simulink model "PosControl_Sim"  (R2017b)
settings: Solver=ode4  StartTime=0.0  StopTime=2  FixedStep=0.001  RelTol=1e-3
InitFcn:
  | Init_control;
values from neighbouring files (symbols this model uses):
  DEG2RAD = 0.0174533    [Init_control.m]
  Kd_PITCH_AngleRate = 0.001    [Init_control.m]
  Kd_ROLL_AngleRate = 0.001    [Init_control.m]
  Kd_YAW_AngleRate = 0.00    (= 0)    [Init_control.m]
  Ki_PITCH_AngleRate = 0.02    [Init_control.m]
  Ki_ROLL_AngleRate = 0.02    [Init_control.m]
  Ki_YAW_AngleRate = 0.01    [Init_control.m]
  Kp_PITCH_ANGLE = 6.5    [Init_control.m]
  Kp_PITCH_AngleRate = 0.1    [Init_control.m]
  Kp_ROLL_ANGLE = 6.5    [Init_control.m]
  Kp_ROLL_AngleRate = 0.1    [Init_control.m]
  Kp_YAW_AngleRate = 0.5    [Init_control.m]
  Kpxp = 1.0    (= 1)    [Init_control.m]
  Kpyp = 1.0    (= 1)    [Init_control.m]
  Kpzp = 4.0    (= 4)    [Init_control.m]
  Kvxd = 0.01    [Init_control.m]
  Kvxi = 0.4    [Init_control.m]
  Kvxp = 2.5    [Init_control.m]
  Kvyd = 0.01    [Init_control.m]
  Kvyi = 0.4    [Init_control.m]
  Kvyp = 2.5    [Init_control.m]
  Kvzd = 0.005    [Init_control.m]
  Kvzi = 0.01    [Init_control.m]
  Kvzp = 0.45    [Init_control.m]
  MAX_CONTROL_ANGLE_PITCH = 35    [Init_control.m]
  MAX_CONTROL_ANGLE_RATE_PITCH = 220    [Init_control.m]
  MAX_CONTROL_ANGLE_RATE_ROLL = 220    [Init_control.m]
  MAX_CONTROL_ANGLE_RATE_Y = 200    [Init_control.m]
  MAX_CONTROL_ANGLE_ROLL = 35    [Init_control.m]
  MAX_CONTROL_VELOCITY_XY = 5    [Init_control.m]
  MAX_CONTROL_VELOCITY_Z = 3    [Init_control.m]
  ModelInit_AngEuler = [0, 0, 0]    [Init_control.m]
  ModelInit_PosE = [0, 0, -100]    [Init_control.m]
  ModelInit_Rads = 0    [Init_control.m]
  ModelInit_RateB = [0, 0, 0]    [Init_control.m]
  ModelInit_VelB = [0, 0, 0]    [Init_control.m]
  Saturation_I_ah = 3.43    [Init_control.m]
  Saturation_I_az = 5    [Init_control.m]
  Saturation_I_RP_Max = 0.3    [Init_control.m]
  Saturation_I_RP_Min = -0.3    [Init_control.m]
  Saturation_I_Y_Max = 0.2    [Init_control.m]
  Saturation_I_Y_Min = -0.2    [Init_control.m]
  THR_HOVER = 0.609    [Init_control.m]
undefined symbols (not defined in the file or in its folder): DiscIntNeverNeededParam, earthRadius, ModelParam_envGravityAcc, ModelParam_motorCr, ModelParam_motorJm, ModelParam_motorT, ModelParam_motorWb, ModelParam_rotorCm, ModelParam_rotorCt, ModelParam_uavCCm, ModelParam_uavCd, ModelParam_uavJ, ModelParam_uavMass, ModelParam_uavR, Receive, Send
libraries: simulink x8, aerolibfltsims x3, sharedutil x2, aerolibanimutils x1
(part 1 of 2)
settings Model: Creator=wsh  LastModifiedBy=Mr Wang
settings DebuggingCC: BusObjectLabelMismatch=error
settings CodeAppCC: StateflowObjectComments=on

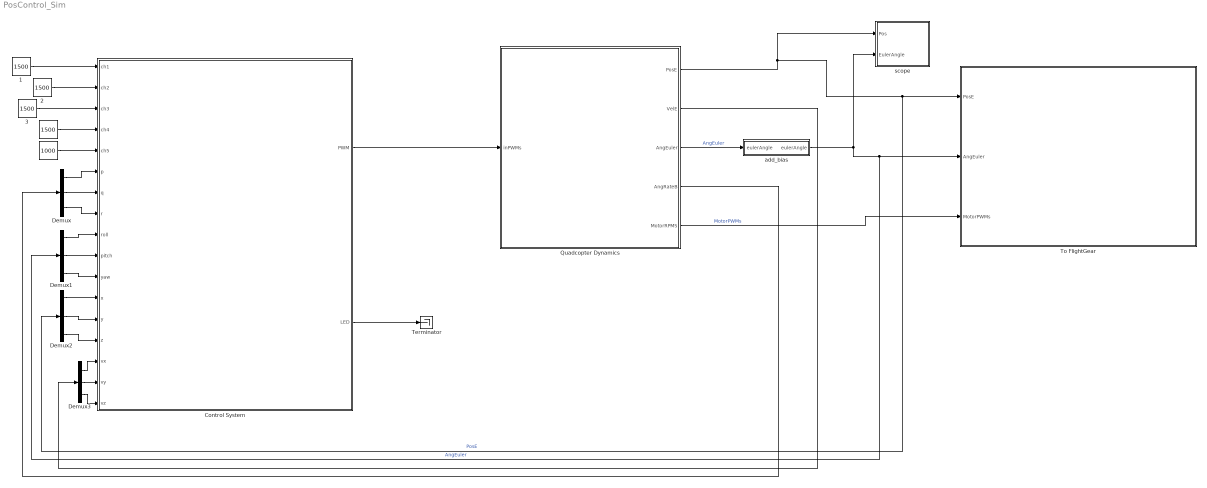
== system PosControl_Sim ==
  " " : Constant  Value=1000  OutDataTypeStr=uint16
  "          " : Constant  Value=1500  OutDataTypeStr=uint16
  "   1" : Constant  Value=1500  OutDataTypeStr=uint16
  "   2" : Constant  Value=1500  OutDataTypeStr=uint16
  "   3" : Constant  Value=1500  OutDataTypeStr=uint16
  Control System : Subsystem
      mask Display: image('icon\pixhawk.png');
  Demux{,1..3} (4 alike) : Demux  Outputs=3
  Quadcopter Dynamics : Subsystem
      mask Display: image('./icon/F450.png');
  Terminator : Terminator
  To FlightGear : Subsystem
      mask Display: image('./icon/FlightGear.png');
  add_bias : Subsystem
  scope : Subsystem
  wires:
  Quadcopter Dynamics/1(PosE) -> scope/1(Pos), To FlightGear/1(PosE), Demux2/1  "PosE"
  Quadcopter Dynamics/5(MotorRPMS) -> To FlightGear/3(MotorPWMs)  "MotorPWMs"
  Control System/2(LED) -> Terminator/1
  add_bias/1("eulerAngle ") -> scope/2(EulerAngle), To FlightGear/2(AngEuler), Demux1/1  "AngEuler"
  "          "/1 -> Control System/4(ch4)
  Quadcopter Dynamics/4(AngRateB) -> Demux/1
  " "/1 -> Control System/5(ch5)
  Demux/1 -> Control System/6(p)
  Demux/2 -> Control System/7(q)
  Demux/3 -> Control System/8(r)
  Demux2/1 -> Control System/12(x)
  Demux2/2 -> Control System/13(y)
  Demux2/3 -> Control System/14(z)
  Demux3/1 -> Control System/15(vx)
  Demux3/2 -> Control System/16(vy)
  Demux3/3 -> Control System/17(vz)
  "   1"/1 -> Control System/1(ch1)
  Quadcopter Dynamics/2(VelE) -> Demux3/1
  "   2"/1 -> Control System/2(ch2)
  Quadcopter Dynamics/3(AngEuler) -> add_bias/1(eulerAngle)  "AngEuler"
  Demux1/2 -> Control System/10(pitch)
  Demux1/1 -> Control System/9(roll)
  Demux1/3 -> Control System/11(yaw)
  "   3"/1 -> Control System/3(ch3)
  Control System/1(PWM) -> Quadcopter Dynamics/1(inPWMs)

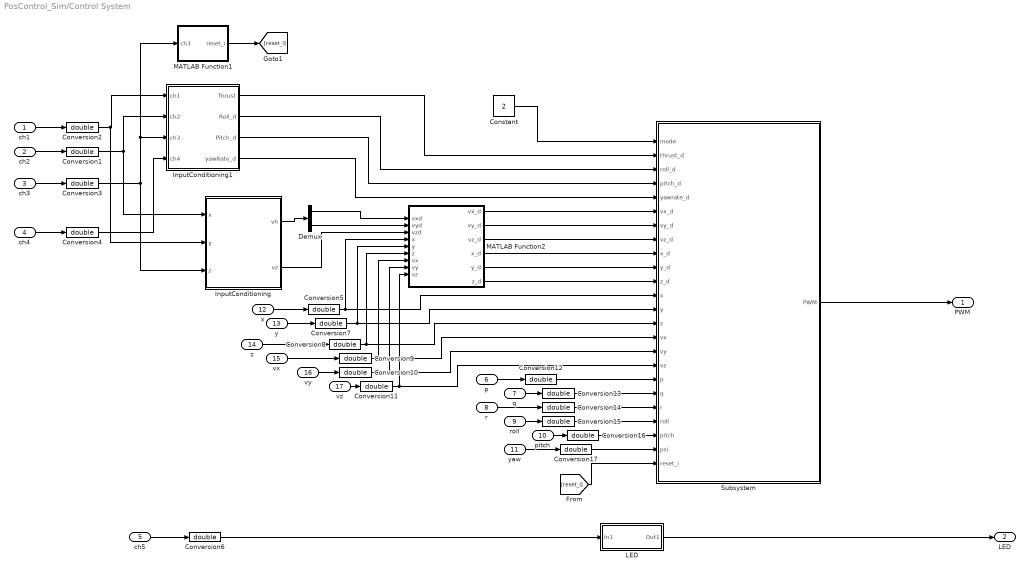
== system PosControl_Sim/Control System ==
  ch1 : Inport  OutDataTypeStr=uint16  PortDimensions=1
  ch2 : Inport  Port=2  OutDataTypeStr=uint16  PortDimensions=1
  ch3 : Inport  Port=3  OutDataTypeStr=uint16  PortDimensions=1
  ch4 : Inport  Port=4  OutDataTypeStr=uint16  PortDimensions=1
  ch5 : Inport  Port=5  OutDataTypeStr=uint16  PortDimensions=1  Interpolate=off
  p : Inport  Port=6  PortDimensions=1
  q : Inport  Port=7  PortDimensions=1
  r : Inport  Port=8  PortDimensions=1
  roll : Inport  Port=9  PortDimensions=1
  pitch : Inport  Port=10  PortDimensions=1
  yaw : Inport  Port=11  PortDimensions=1
  x : Inport  Port=12
  y : Inport  Port=13
  z : Inport  Port=14
  vx : Inport  Port=15
  vy : Inport  Port=16
  vz : Inport  Port=17
  Constant : Constant  Value=2
  Conversion{1..17} (17 alike) : DataTypeConversion  OutDataTypeStr=double
  Demux : Demux  Outputs=2
  InputConditioning : Subsystem
  InputConditioning1 : Subsystem
  "LED " : Subsystem
  MATLAB Function1 : MATLAB Function  TreatAsAtomicUnit=on
  MATLAB Function2 : MATLAB Function  TreatAsAtomicUnit=on
  Subsystem : Subsystem
  PWM : Outport
  LED : Outport  Port=2  PortDimensions=1
  wires:
  ch3/1 -> Conversion3/1
  ch5/1 -> Conversion6/1
  ch4/1 -> Conversion4/1
  "LED "/1(Out1) -> LED/1
  Conversion6/1 -> "LED "/1(In1)
  Conversion4/1 -> InputConditioning1/4(ch4)
  ch1/1 -> Conversion2/1
  ch2/1 -> Conversion1/1
  Conversion1/1 -> InputConditioning/1(x), InputConditioning1/2(ch2)
  x/1 -> Conversion5/1
  y/1 -> Conversion7/1
  z/1 -> Conversion8/1
  Constant/1 -> Subsystem/1(mode)
  roll/1 -> Conversion15/1
  pitch/1 -> Conversion16/1
  p/1 -> Conversion12/1
  q/1 -> Conversion13/1
  r/1 -> Conversion14/1
  yaw/1 -> Conversion17/1
  vz/1 -> Conversion11/1
  vy/1 -> Conversion10/1
  vx/1 -> Conversion9/1
  InputConditioning1/2(Roll_d) -> Subsystem/3(roll_d)
  InputConditioning1/3(Pitch_d) -> Subsystem/4(pitch_d)
  InputConditioning1/1(Thrust) -> Subsystem/2(thrust_d)
  InputConditioning1/4(yawRate_d) -> Subsystem/5(yawrate_d)
  Conversion5/1 -> Subsystem/12(x), MATLAB Function2/4(x)
  Conversion7/1 -> Subsystem/13(y), MATLAB Function2/5(y)
  Conversion8/1 -> Subsystem/14(z), MATLAB Function2/6(z)
  Conversion9/1 -> Subsystem/15(vx), MATLAB Function2/7(vx)
  Conversion10/1 -> Subsystem/16(vy), MATLAB Function2/8(vy)
  Conversion11/1 -> Subsystem/17(vz), MATLAB Function2/9(vz)
  Conversion12/1 -> Subsystem/18(p)
  Conversion13/1 -> Subsystem/19(q)
  Conversion14/1 -> Subsystem/20(r)
  Conversion15/1 -> Subsystem/21(roll)
  Conversion16/1 -> Subsystem/22(pitch)
  Conversion17/1 -> Subsystem/23(psi)
  Conversion3/1 -> InputConditioning/3(z), InputConditioning1/3(ch3), MATLAB Function1/1(ch3)
  MATLAB Function1/1(reset_i) -> [reset_i]
  [reset_i] -> Subsystem/24(reset_i)
  Conversion2/1 -> InputConditioning/2(y), InputConditioning1/1("ch1 ")
  InputConditioning/2(vz) -> MATLAB Function2/3(vzd)
  MATLAB Function2/1(vx_d) -> Subsystem/6(vx_d)
  MATLAB Function2/2(vy_d) -> Subsystem/7(vy_d)
  MATLAB Function2/3(vz_d) -> Subsystem/8(vz_d)
  MATLAB Function2/4(x_d) -> Subsystem/9(x_d)
  MATLAB Function2/5(y_d) -> Subsystem/10(y_d)
  MATLAB Function2/6(z_d) -> Subsystem/11(z_d)
  InputConditioning/1(vh) -> Demux/1
  Demux/1 -> MATLAB Function2/1(vxd)
  Demux/2 -> MATLAB Function2/2(vyd)
  Subsystem/1(PWM) -> PWM/1

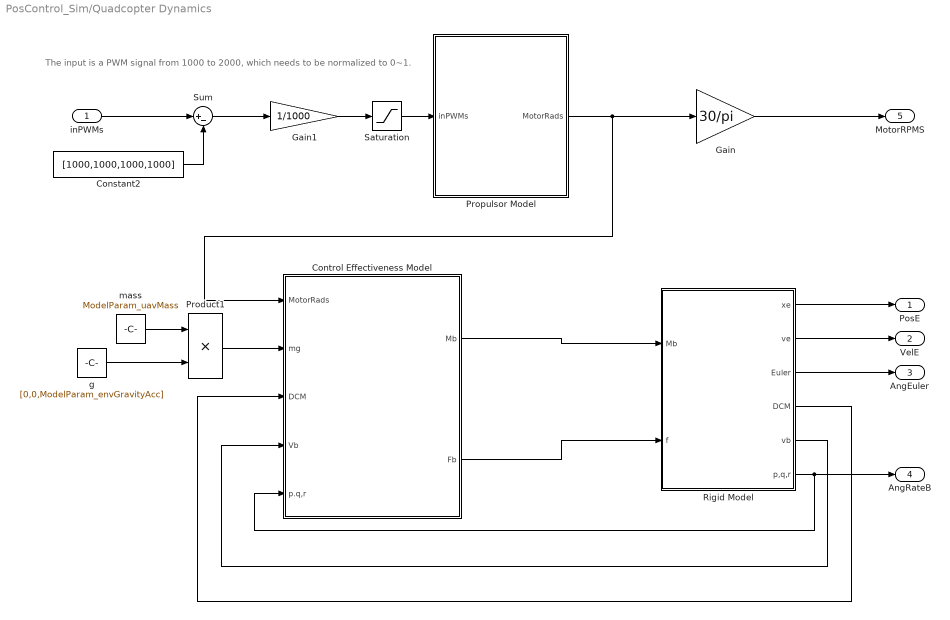
== system PosControl_Sim/Quadcopter Dynamics ==
  note: The input is a PWM signal from 1000 to 2000,
      | which needs to be normalized to 0~1.
  inPWMs : Inport
  Constant2 : Constant  Value=[1000,1000,1000,1000]
  Control Effectiveness Model : Subsystem
  Gain : Gain  Gain=30/pi
  Gain1 : Gain  Gain=1/1000
  Product1 : Product
  Propulsor Model : Subsystem
  Rigid Model : Subsystem
  Saturation : Saturate  UpperLimit=1  LowerLimit=0
  Sum : Sum  Inputs=|+-
  g : Constant  Value=[0,0,ModelParam_envGravityAcc]
  mass : Constant  Value=ModelParam_uavMass
  PosE : Outport
  VelE : Outport  Port=2
  AngEuler : Outport  Port=3
  AngRateB : Outport  Port=4
  MotorRPMS : Outport  Port=5
  wires:
  Saturation/1 -> Propulsor Model/1(inPWMs)
  Rigid Model/6("p,q,r ") -> Control Effectiveness Model/5(p.q,r), AngRateB/1
  mass/1 -> Product1/1
  Rigid Model/4(DCM) -> Control Effectiveness Model/3(DCM)
  Propulsor Model/1(MotorRads) -> Gain/1, Control Effectiveness Model/1(MotorRads)
  Gain1/1 -> Saturation/1
  Rigid Model/2(ve) -> VelE/1
  Sum/1 -> Gain1/1
  Product1/1 -> Control Effectiveness Model/2(mg)
  Rigid Model/5("vb ") -> Control Effectiveness Model/4(Vb)
  Rigid Model/1("xe ") -> PosE/1
  Rigid Model/3(Euler) -> AngEuler/1
  Control Effectiveness Model/1(Mb) -> Rigid Model/1(Mb)
  inPWMs/1 -> Sum/1
  Control Effectiveness Model/2(Fb) -> Rigid Model/2(f)
  Constant2/1 -> Sum/2
  g/1 -> Product1/2
  Gain/1 -> MotorRPMS/1

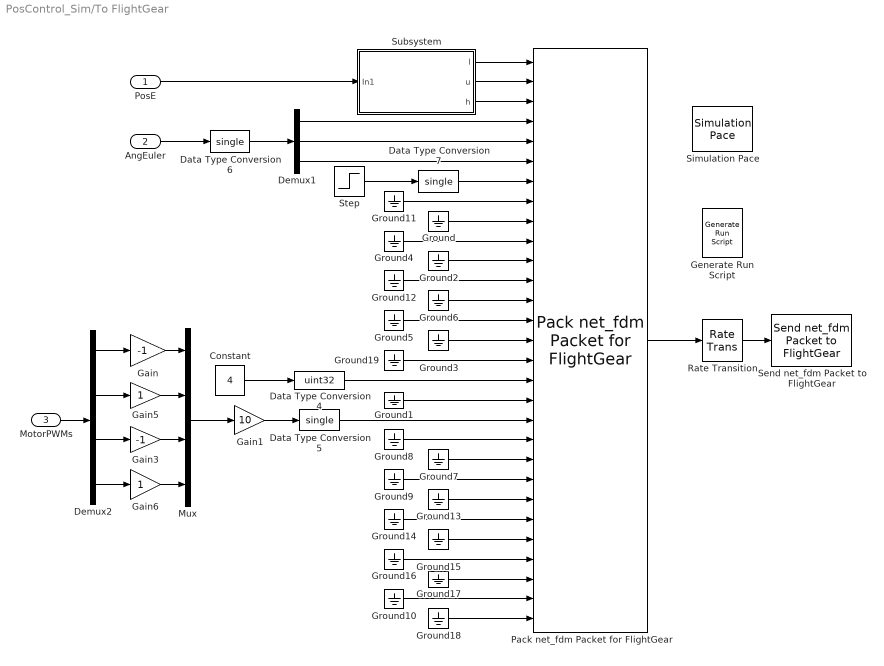
== system PosControl_Sim/To FlightGear ==
  PosE : Inport
  AngEuler : Inport  Port=2
  MotorPWMs : Inport  Port=3
  Constant : Constant  Value=4
  Data Type Conversion4 : DataTypeConversion  OutDataTypeStr=uint32
  Data Type Conversion5 : DataTypeConversion  OutDataTypeStr=single
  Data Type Conversion6 : DataTypeConversion  OutDataTypeStr=single
  Data Type Conversion7 : DataTypeConversion  OutDataTypeStr=single
  Demux1 : Demux  Outputs=3
  Demux2 : Demux
  Gain : Gain  Gain=-1
  Gain1 : Gain  Gain=10
  Gain3 : Gain  Gain=-1
  Gain5 : Gain
  Gain6 : Gain
  Generate Run Script : aerolibfltsims/Generate Run Script  OutputFileName=runfg_myownUAV.bat  FlightGearBaseDirectory=C:\Program Files\FlightGear 2016.1.2  GeometryModelName=myownUAV  DestinationPort=5502  OriginAddress=127.0.0.1  OriginPort=5505  LocalAddress=127.0.0.1  AirportId=KSFO  RunwayId=10L  InitialAltitude=0  InitialHeading=0  OffsetDistance=0  OffsetAzimuth=0  GenerateFile=off  Architecture=Default  dataFlow=Send-Receive
  Ground{,1..19} (20 alike) : Ground
  Mux : Mux
  Pack net_fdm Packet for FlightGear : aerolibfltsims/Pack net_fdm Packet for FlightGear  FlightGearVersion=v2016.1  ShowPositionAttitudeInputs=on  ShowVelocityAccelerationInputs=off  ShowControlSurfacePositionInputs=on  ShowEngineFuelInputs=on  ShowLandingGearInputs=off  ShowEnvironmentInputs=off  SampleTime=0.01
      settings: SourceProductName=Aerospace Blockset  SourceProductBaseCode=AE
  Rate Transition : RateTransition
  Send net_fdm Packet to FlightGear : aerolibfltsims/Send net_fdm Packet to FlightGear  DestinationIpAddress=127.0.0.1  DestinationPort=5502  LocalIpPort=-1  varLen=off  SampleTime=0.005
      settings: SourceProductName=Aerospace Blockset  SourceProductBaseCode=AE
  Simulation Pace : aerolibanimutils/Simulation Pace  SimulationPace=1  SleepMode=MATLAB Thread  OutputPaceError=off  SampleTime=-1
      settings: AttributesFormatString=%<SimulationPace> sec/sec
  Step : Step  Time=0  SampleTime=0
  Subsystem : Subsystem
  wires:
  Gain1/1 -> Data Type Conversion5/1
  Data Type Conversion6/1 -> Demux1/1
  Demux1/3 -> Pack net_fdm Packet for FlightGear/6
  Demux1/2 -> Pack net_fdm Packet for FlightGear/5
  Demux1/1 -> Pack net_fdm Packet for FlightGear/4
  Ground19/1 -> Pack net_fdm Packet for FlightGear/16
  Subsystem/3(h) -> Pack net_fdm Packet for FlightGear/3
  Subsystem/2(u) -> Pack net_fdm Packet for FlightGear/2
  Subsystem/1("l ") -> Pack net_fdm Packet for FlightGear/1
  PosE/1 -> Subsystem/1(In1)
  Rate Transition/1 -> Send net_fdm Packet to FlightGear/1
  Gain6/1 -> Mux/4
  Demux2/4 -> Gain6/1
  Gain5/1 -> Mux/2
  Demux2/2 -> Gain5/1
  Gain3/1 -> Mux/3
  Gain/1 -> Mux/1
  Demux2/3 -> Gain3/1
  Demux2/1 -> Gain/1
  Mux/1 -> Gain1/1
  MotorPWMs/1 -> Demux2/1
  AngEuler/1 -> Data Type Conversion6/1
  Ground12/1 -> Pack net_fdm Packet for FlightGear/12
  Ground2/1 -> Pack net_fdm Packet for FlightGear/11
  Data Type Conversion5/1 -> Pack net_fdm Packet for FlightGear/19
  Constant/1 -> Data Type Conversion4/1
  Ground11/1 -> Pack net_fdm Packet for FlightGear/8
  Ground4/1 -> Pack net_fdm Packet for FlightGear/10
  Ground6/1 -> Pack net_fdm Packet for FlightGear/13
  Ground5/1 -> Pack net_fdm Packet for FlightGear/14
  Ground3/1 -> Pack net_fdm Packet for FlightGear/15
  Ground1/1 -> Pack net_fdm Packet for FlightGear/18
  Data Type Conversion4/1 -> Pack net_fdm Packet for FlightGear/17
  Step/1 -> Data Type Conversion7/1
  Ground18/1 -> Pack net_fdm Packet for FlightGear/29
  Ground10/1 -> Pack net_fdm Packet for FlightGear/28
  Ground17/1 -> Pack net_fdm Packet for FlightGear/27
  Ground16/1 -> Pack net_fdm Packet for FlightGear/26
  Ground15/1 -> Pack net_fdm Packet for FlightGear/25
  Ground14/1 -> Pack net_fdm Packet for FlightGear/24
  Ground13/1 -> Pack net_fdm Packet for FlightGear/23
  Ground9/1 -> Pack net_fdm Packet for FlightGear/22
  Ground7/1 -> Pack net_fdm Packet for FlightGear/21
  Ground/1 -> Pack net_fdm Packet for FlightGear/9
  Ground8/1 -> Pack net_fdm Packet for FlightGear/20
  Data Type Conversion7/1 -> Pack net_fdm Packet for FlightGear/7
  Pack net_fdm Packet for FlightGear/1 -> Rate Transition/1

== system PosControl_Sim/add_bias ==
  eulerAngle : Inport
  Constant : Constant  Value=0.03
  Constant1 : Constant  Value=0.03
  Demux4 : Demux  Outputs=3
  Mux : Mux  Inputs=3
  Sum : Sum  Inputs=|++
  Sum1 : Sum  Inputs=|++
  "eulerAngle " : Outport
  wires:
  Sum/1 -> Mux/1
  eulerAngle/1 -> Demux4/1
  Sum1/1 -> Mux/2
  Demux4/3 -> Mux/3  "yaw"
  Demux4/2 -> Sum1/1  "pitch"
  Constant/1 -> Sum/2
  Demux4/1 -> Sum/1  "roll"
  Constant1/1 -> Sum1/2
  Mux/1 -> "eulerAngle "/1

== system PosControl_Sim/scope ==
  Pos : Inport
  EulerAngle : Inport  Port=2
  Demux1 : Demux  Outputs=3
  Demux4 : Demux  Outputs=3
  Terminator : Terminator
  XY : simulink/Sinks/XY Graph  xmin=-0.2  xmax=3  ymin=-3  ymax=0.2  st=-1
  rp : Scope  NumInputPorts=2
  z : Scope
  wires:
  Demux1/1 -> XY/1
  Demux4/2 -> rp/2
  Demux4/1 -> rp/1
  Demux4/3 -> Terminator/1
  EulerAngle/1 -> Demux4/1
  Pos/1 -> Demux1/1
  Demux1/3 -> z/1
  Demux1/2 -> XY/2

== system PosControl_Sim/Control System/InputConditioning ==
  x : Inport
  y : Inport  Port=2
  z : Inport  Port=3
  Mux21 : Mux  Inputs=2
  Saturation10 : Saturate  UpperLimit=1  LowerLimit=-1
  Saturation8 : Saturate  UpperLimit=1  LowerLimit=-1
  Saturation9 : Saturate  UpperLimit=1  LowerLimit=-1
  deadzone1 : MATLAB Function  TreatAsAtomicUnit=on
  deadzone2 : MATLAB Function  TreatAsAtomicUnit=on
  deadzone3 : MATLAB Function  TreatAsAtomicUnit=on
  max_vx : Gain  Gain=-MAX_CONTROL_VELOCITY_XY  OutDataTypeStr=Inherit: Inherit via back propagation
  max_vy : Gain  Gain=MAX_CONTROL_VELOCITY_XY  OutDataTypeStr=Inherit: Inherit via back propagation
  max_vz : Gain  Gain=-MAX_CONTROL_VELOCITY_Z  OutDataTypeStr=Inherit: Inherit via back propagation
  vh : Outport
  vz : Outport  Port=2
  wires:
  Saturation10/1 -> max_vz/1
  Mux21/1 -> vh/1
  Saturation8/1 -> max_vx/1
  deadzone3/1(y) -> Saturation10/1
  deadzone2/1(y) -> Saturation9/1
  deadzone1/1(y) -> Saturation8/1
  Saturation9/1 -> max_vy/1
  x/1 -> deadzone1/1(u)
  z/1 -> deadzone3/1(u)
  y/1 -> deadzone2/1(u)
  max_vz/1 -> vz/1
  max_vx/1 -> Mux21/1
  max_vy/1 -> Mux21/2

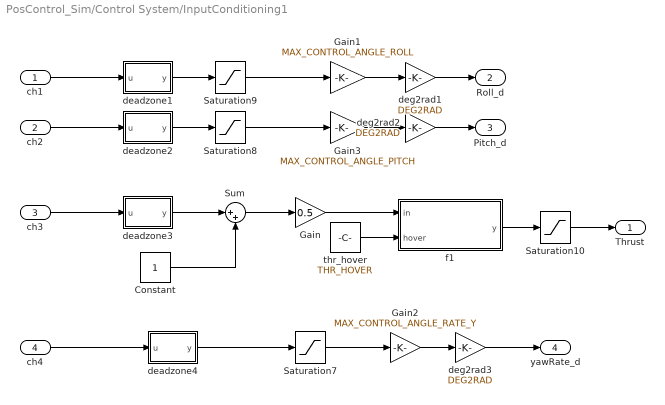
== system PosControl_Sim/Control System/InputConditioning1 ==
  "ch1 " : Inport
  ch2 : Inport  Port=2
  ch3 : Inport  Port=3
  ch4 : Inport  Port=4
  Constant : Constant
  Gain : Gain  Gain=0.5
  Gain1 : Gain  Gain=MAX_CONTROL_ANGLE_ROLL  OutDataTypeStr=Inherit: Inherit via back propagation
  Gain2 : Gain  Gain=MAX_CONTROL_ANGLE_RATE_Y
  Gain3 : Gain  Gain=MAX_CONTROL_ANGLE_PITCH  OutDataTypeStr=Inherit: Inherit via back propagation
  Saturation10 : Saturate  UpperLimit=1  LowerLimit=0
  Saturation7 : Saturate  UpperLimit=1  LowerLimit=-1
  Saturation8 : Saturate  UpperLimit=1  LowerLimit=-1
  Saturation9 : Saturate  UpperLimit=1  LowerLimit=-1
  Sum : Sum  Inputs=|++
  deadzone1 : MATLAB Function  TreatAsAtomicUnit=on
  deadzone2 : MATLAB Function  TreatAsAtomicUnit=on
  deadzone3 : MATLAB Function  TreatAsAtomicUnit=on
  deadzone4 : MATLAB Function  TreatAsAtomicUnit=on
  deg2rad1 : Gain  Gain=DEG2RAD
  deg2rad2 : Gain  Gain=DEG2RAD
  deg2rad3 : Gain  Gain=DEG2RAD
  f1 : MATLAB Function  TreatAsAtomicUnit=on
  "thr_hover " : Constant  Value=THR_HOVER
  Thrust : Outport
  Roll_d : Outport  Port=2
  Pitch_d : Outport  Port=3
  yawRate_d : Outport  Port=4
  wires:
  deadzone3/1(y) -> Sum/1
  ch3/1 -> deadzone3/1(u)
  deadzone2/1(y) -> Saturation8/1
  Saturation10/1 -> Thrust/1
  deadzone1/1(y) -> Saturation9/1
  "ch1 "/1 -> deadzone1/1(u)
  ch2/1 -> deadzone2/1(u)
  Saturation9/1 -> Gain1/1
  Saturation8/1 -> Gain3/1
  Gain3/1 -> deg2rad2/1
  Constant/1 -> Sum/2
  Sum/1 -> Gain/1
  Gain1/1 -> deg2rad1/1
  deg2rad1/1 -> Roll_d/1
  deg2rad2/1 -> Pitch_d/1
  Saturation7/1 -> Gain2/1
  deadzone4/1(y) -> Saturation7/1
  ch4/1 -> deadzone4/1(u)
  Gain2/1 -> deg2rad3/1
  deg2rad3/1 -> yawRate_d/1
  "thr_hover "/1 -> f1/2(hover)
  Gain/1 -> f1/1(in)
  f1/1(y) -> Saturation10/1

== system PosControl_Sim/Control System/LED  ==
  In1 : Inport
  Compare To Constant3 : simulink/Logic and Bit Operations/Compare To Constant  relop=>=  const=uint16(1500)  OutDataTypeStr=boolean
  Out1 : Outport
  wires:
  Compare To Constant3/1 -> Out1/1
  In1/1 -> Compare To Constant3/1

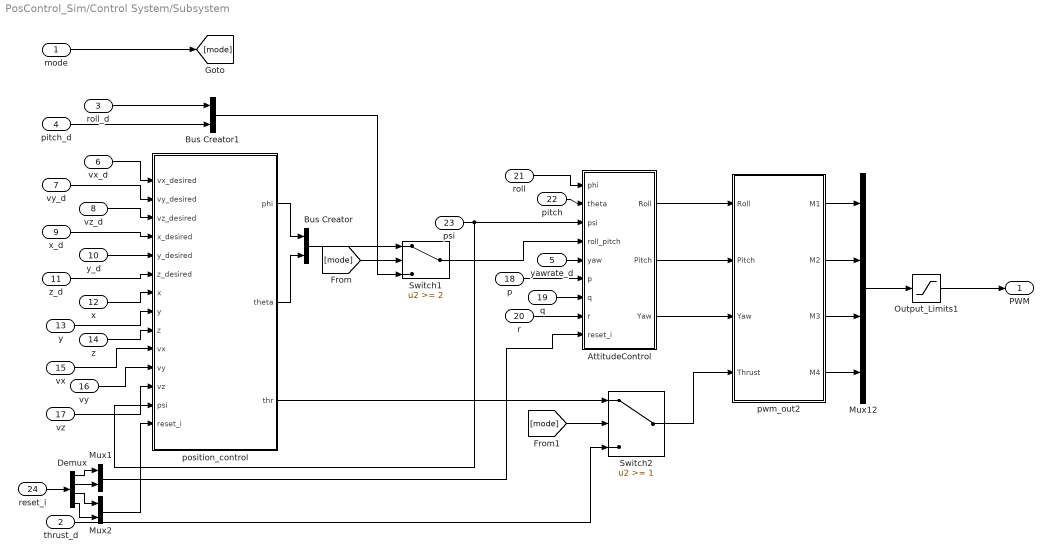
== system PosControl_Sim/Control System/Subsystem ==
  mode : Inport
  thrust_d : Inport  Port=2
  roll_d : Inport  Port=3
  pitch_d : Inport  Port=4
  yawrate_d : Inport  Port=5
  vx_d : Inport  Port=6
  vy_d : Inport  Port=7
  vz_d : Inport  Port=8
  x_d : Inport  Port=9
  y_d : Inport  Port=10
  z_d : Inport  Port=11
  x : Inport  Port=12
  y : Inport  Port=13
  z : Inport  Port=14
  vx : Inport  Port=15
  vy : Inport  Port=16
  vz : Inport  Port=17
  p : Inport  Port=18  PortDimensions=1
  q : Inport  Port=19  PortDimensions=1
  r : Inport  Port=20  PortDimensions=1
  roll : Inport  Port=21  PortDimensions=1
  pitch : Inport  Port=22  PortDimensions=1
  psi : Inport  Port=23  PortDimensions=1
  reset_i : Inport  Port=24
  AttitudeControl : Subsystem
  Bus Creator : BusCreator  Inputs=2
  Bus Creator1 : BusCreator  Inputs=2
  Demux : Demux
  Mux1 : Mux  Inputs=2
  Mux12 : Mux
  Mux2 : Mux  Inputs=2
  Output_Limits1 : Saturate  UpperLimit=2000  LowerLimit=1000
  Switch1 : Switch  Threshold=2
  Switch2 : Switch  Threshold=1
  position_control : Subsystem
  pwm_out2 : MATLAB Function  SystemSampleTime=0.004
  PWM : Outport
  wires:
  pwm_out2/4(M4) -> Mux12/4
  pwm_out2/3(M3) -> Mux12/3
  yawrate_d/1 -> AttitudeControl/5(yaw)
  roll/1 -> AttitudeControl/1(phi)
  Output_Limits1/1 -> PWM/1
  q/1 -> AttitudeControl/7(q)
  AttitudeControl/1(Roll) -> pwm_out2/1(Roll)
  pwm_out2/2(M2) -> Mux12/2
  AttitudeControl/2(Pitch) -> pwm_out2/2(Pitch)
  pitch/1 -> AttitudeControl/2(theta)
  Mux12/1 -> Output_Limits1/1
  position_control/2(theta) -> Bus Creator/2
  pwm_out2/1(M1) -> Mux12/1
  AttitudeControl/3(Yaw) -> pwm_out2/3(Yaw)
  position_control/1(phi) -> Bus Creator/1
  p/1 -> AttitudeControl/6(p)
  vx/1 -> position_control/10(vx)
  vz/1 -> position_control/12(vz)
  vy/1 -> position_control/11(vy)
  x_d/1 -> position_control/4(x_desired)
  y_d/1 -> position_control/5(y_desired)
  z_d/1 -> position_control/6(z_desired)
  mode/1 -> [mode]
  vz_d/1 -> position_control/3(vz_desired)
  x/1 -> position_control/7(x)
  vx_d/1 -> position_control/1(vx_desired)
  vy_d/1 -> position_control/2(vy_desired)
  y/1 -> position_control/8(y)
  z/1 -> position_control/9(z)
  Bus Creator/1 -> Switch1/1
  [mode] -> Switch1/2
  Switch1/1 -> AttitudeControl/4(roll_pitch)
  roll_d/1 -> Bus Creator1/1
  pitch_d/1 -> Bus Creator1/2
  Bus Creator1/1 -> Switch1/3
  [mode] -> Switch2/2
  position_control/3(thr) -> Switch2/1
  Switch2/1 -> pwm_out2/4(Thrust)
  thrust_d/1 -> Switch2/3
  r/1 -> AttitudeControl/8(r)
  psi/1 -> AttitudeControl/3(psi), position_control/13(psi)
  reset_i/1 -> Demux/1
  Mux2/1 -> position_control/14(reset_i)
  Mux1/1 -> AttitudeControl/9(reset_i)
  Demux/1 -> Mux1/1
  Demux/2 -> Mux1/2
  Demux/3 -> Mux2/1
  Demux/4 -> Mux2/2

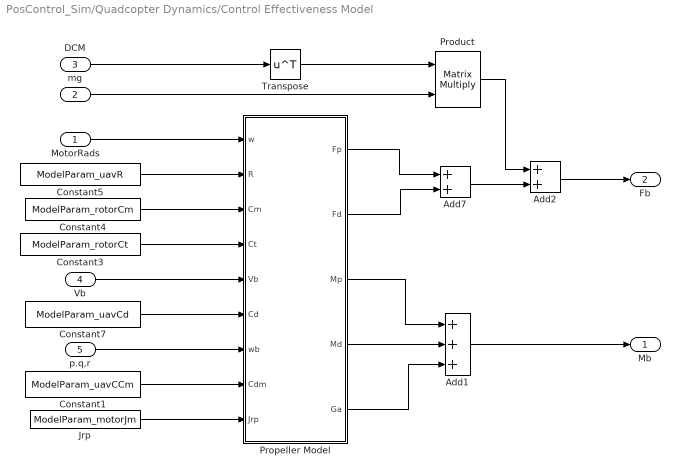
== system PosControl_Sim/Quadcopter Dynamics/Control Effectiveness Model ==
  MotorRads : Inport
  mg : Inport  Port=2
  DCM : Inport  Port=3
  Vb : Inport  Port=4
  p.q,r : Inport  Port=5
  Add1 : Sum  Inputs=+++
  Add2 : Sum
  Add7 : Sum
  Constant1 : Constant  Value=ModelParam_uavCCm
  Constant3 : Constant  Value=ModelParam_rotorCt
  Constant4 : Constant  Value=ModelParam_rotorCm
  Constant5 : Constant  Value=ModelParam_uavR
  Constant7 : Constant  Value=ModelParam_uavCd
  Jrp : Constant  Value=ModelParam_motorJm
  Product : Product  Multiplication=Matrix(*)
  Propeller Model : MATLAB Function  TreatAsAtomicUnit=on
  Transpose : Math  Operator=transpose  SaturateOnIntegerOverflow=on
  Mb : Outport
  Fb : Outport  Port=2
  wires:
  Add2/1 -> Fb/1
  Constant3/1 -> Propeller Model/4(Ct)
  Propeller Model/2(Fd) -> Add7/2
  Add7/1 -> Add2/2
  Propeller Model/1(Fp) -> Add7/1
  Product/1 -> Add2/1
  mg/1 -> Product/2
  DCM/1 -> Transpose/1
  Constant7/1 -> Propeller Model/6(Cd)
  Vb/1 -> Propeller Model/5(Vb)
  Constant5/1 -> Propeller Model/2(R)
  Constant4/1 -> Propeller Model/3(Cm)
  MotorRads/1 -> Propeller Model/1(w)
  Transpose/1 -> Product/1
  Propeller Model/3(Mp) -> Add1/1
  Propeller Model/4(Md) -> Add1/2
  Add1/1 -> Mb/1
  p.q,r/1 -> Propeller Model/7(wb)
  Constant1/1 -> Propeller Model/8(Cdm)
  Jrp/1 -> Propeller Model/9(Jrp)
  Propeller Model/5(Ga) -> Add1/3

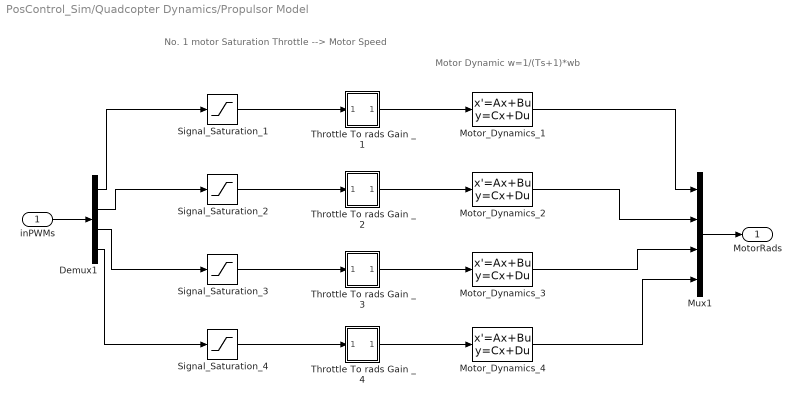
== system PosControl_Sim/Quadcopter Dynamics/Propulsor Model ==
  note: Motor Dynamic
      | w=1/(Ts+1)*wb
  note: No. 1 motor
      |
      |          Saturation             Throttle --> Motor Speed
  inPWMs : Inport
  Demux1 : Demux
  Motor_Dynamics_{1..4} (4 alike) : StateSpace  A=-1/ModelParam_motorT  C=1/ModelParam_motorT  D=0  InitialCondition=ModelInit_Rads*ModelParam_motorT
  Mux1 : Mux
  Signal_Saturation_{1..4} (4 alike) : Saturate  UpperLimit=1  LowerLimit=0
  Throttle To rads Gain _1 : Subsystem
  Throttle To rads Gain _2 : Subsystem
  Throttle To rads Gain _3 : Subsystem
  Throttle To rads Gain _4 : Subsystem
  MotorRads : Outport
  wires:
  Throttle To rads Gain _4/1(Out5) -> Motor_Dynamics_4/1
  Signal_Saturation_4/1 -> Throttle To rads Gain _4/1(In5)
  Signal_Saturation_3/1 -> Throttle To rads Gain _3/1(In5)
  Signal_Saturation_2/1 -> Throttle To rads Gain _2/1(In5)
  Motor_Dynamics_4/1 -> Mux1/4
  Motor_Dynamics_3/1 -> Mux1/3
  Motor_Dynamics_2/1 -> Mux1/2
  Motor_Dynamics_1/1 -> Mux1/1
  Signal_Saturation_1/1 -> Throttle To rads Gain _1/1(In5)
  Mux1/1 -> MotorRads/1
  Throttle To rads Gain _3/1(Out5) -> Motor_Dynamics_3/1
  Throttle To rads Gain _2/1(Out5) -> Motor_Dynamics_2/1
  Throttle To rads Gain _1/1(Out5) -> Motor_Dynamics_1/1
  inPWMs/1 -> Demux1/1
  Demux1/4 -> Signal_Saturation_4/1
  Demux1/3 -> Signal_Saturation_3/1
  Demux1/2 -> Signal_Saturation_2/1
  Demux1/1 -> Signal_Saturation_1/1

== system PosControl_Sim/Quadcopter Dynamics/Rigid Model ==
  Mb : Inport
  f : Inport  Port=2
  Rigid-Body Dynamic Model : Subsystem
  "Rigid-Body Kinematic Model " : Subsystem
  "xe " : Outport
  ve : Outport  Port=2
  Euler : Outport  Port=3
  DCM : Outport  Port=4
  "vb " : Outport  Port=5
  "p,q,r " : Outport  Port=6
  wires:
  Rigid-Body Dynamic Model/1("p,q,r ") -> "Rigid-Body Kinematic Model "/1(pqr), "p,q,r "/1
  "Rigid-Body Kinematic Model "/1(Euler) -> Euler/1
  "Rigid-Body Kinematic Model "/3(DCM) -> Rigid-Body Dynamic Model/3(DCM), DCM/1
  Mb/1 -> Rigid-Body Dynamic Model/1(Mb)
  f/1 -> Rigid-Body Dynamic Model/2(f)
  Rigid-Body Dynamic Model/2(ve) -> "Rigid-Body Kinematic Model "/2(ve), ve/1
  Rigid-Body Dynamic Model/3("vb ") -> "vb "/1
  "Rigid-Body Kinematic Model "/2("xe ") -> "xe "/1

== system PosControl_Sim/To FlightGear/Subsystem ==
  In1 : Inport
  Constant1 : Constant  Value=5  VectorParams1D=off
  Constant2 : Constant  Value=-2.1361  VectorParams1D=off
  Constant3 : Constant  Value=0.65673  VectorParams1D=off
  Demux : Demux  Outputs=3
  Gain1 : Gain  Gain=10/earthRadius
  Gain2 : Gain  Gain=10/earthRadius
  Gain4 : Gain
  Gain8 : Gain  Gain=-10
  Sum10 : Sum  Inputs=|++
  Sum8 : Sum  Inputs=|++
  Sum9 : Sum  Inputs=|++
  "l " : Outport
  u : Outport  Port=2
  h : Outport  Port=3
  wires:
  Sum8/1 -> "l "/1
  In1/1 -> Demux/1
  Sum9/1 -> u/1
  Sum10/1 -> h/1
  Gain4/1 -> Gain2/1
  Demux/2 -> Gain1/1
  Gain8/1 -> Sum10/1
  Gain1/1 -> Sum8/1
  Gain2/1 -> Sum9/1
  Constant2/1 -> Sum8/2
  Demux/3 -> Gain8/1
  Demux/1 -> Gain4/1
  Constant1/1 -> Sum10/2
  Constant3/1 -> Sum9/2

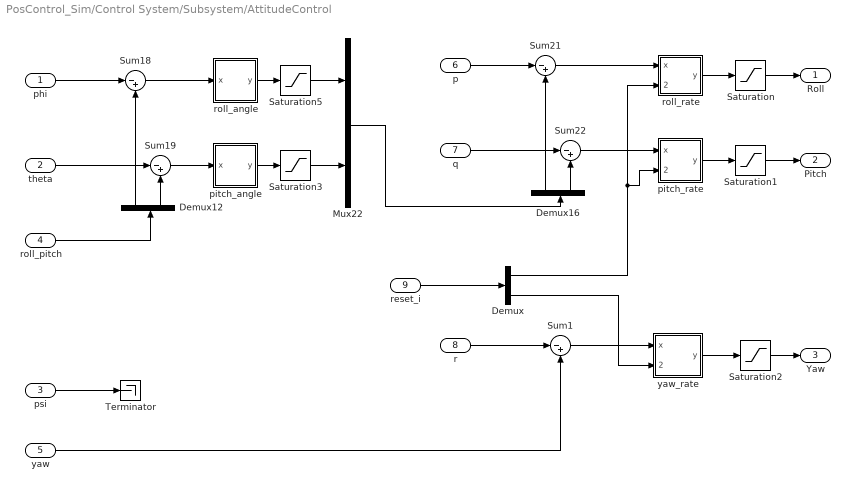
== system PosControl_Sim/Control System/Subsystem/AttitudeControl ==
  phi : Inport
  theta : Inport  Port=2
  psi : Inport  Port=3
  roll_pitch : Inport  Port=4
  yaw : Inport  Port=5
  p : Inport  Port=6
  q : Inport  Port=7
  r : Inport  Port=8
  reset_i : Inport  Port=9
  Demux : Demux  Outputs=2
  Demux12 : Demux  Outputs=2
  Demux16 : Demux  Outputs=2
  Mux22 : Mux  Inputs=2
  Saturation : Saturate  UpperLimit=1  LowerLimit=-1
  Saturation1 : Saturate  UpperLimit=1  LowerLimit=-1
  Saturation2 : Saturate
  Saturation3 : Saturate  UpperLimit=MAX_CONTROL_ANGLE_RATE_PITCH  LowerLimit=-MAX_CONTROL_ANGLE_RATE_PITCH
  Saturation5 : Saturate  UpperLimit=MAX_CONTROL_ANGLE_RATE_ROLL  LowerLimit=-MAX_CONTROL_ANGLE_RATE_ROLL
  Sum1 : Sum  Inputs=|-+
  Sum18 : Sum  Inputs=|-+  OutMin=-90  OutMax=90
  Sum19 : Sum  Inputs=|-+  OutMin=-90  OutMax=90
  Sum21 : Sum  Inputs=|-+
  Sum22 : Sum  Inputs=|-+
  Terminator : Terminator
  "pitch_angle " : Subsystem
  pitch_rate : Subsystem
  "roll_angle " : Subsystem
  roll_rate : Subsystem
  yaw_rate : Subsystem
  Roll : Outport
  Pitch : Outport  Port=2
  Yaw : Outport  Port=3
  wires:
  Sum19/1 -> "pitch_angle "/1(x)
  "pitch_angle "/1(y) -> Saturation3/1
  Demux12/1 -> Sum18/2
  Demux12/2 -> Sum19/2
  phi/1 -> Sum18/1
  theta/1 -> Sum19/1
  Sum18/1 -> "roll_angle "/1(x)
  Sum22/1 -> pitch_rate/1(x)
  p/1 -> Sum21/1
  q/1 -> Sum22/1
  Sum21/1 -> roll_rate/1(x)
  Demux16/1 -> Sum21/2
  pitch_rate/1(y) -> Saturation1/1
  roll_rate/1(y) -> Saturation/1
  yaw_rate/1(y) -> Saturation2/1
  roll_pitch/1 -> Demux12/1
  Saturation/1 -> Roll/1
  Saturation1/1 -> Pitch/1
  Saturation2/1 -> Yaw/1
  Demux16/2 -> Sum22/2
  Mux22/1 -> Demux16/1
  r/1 -> Sum1/1
  Sum1/1 -> yaw_rate/1(x)
  "roll_angle "/1(y) -> Saturation5/1
  Saturation5/1 -> Mux22/1
  Saturation3/1 -> Mux22/2
  yaw/1 -> Sum1/2
  Demux/1 -> roll_rate/2(reset_i), pitch_rate/2(reset_i)
  reset_i/1 -> Demux/1
  Demux/2 -> yaw_rate/2(reset_i)
  psi/1 -> Terminator/1

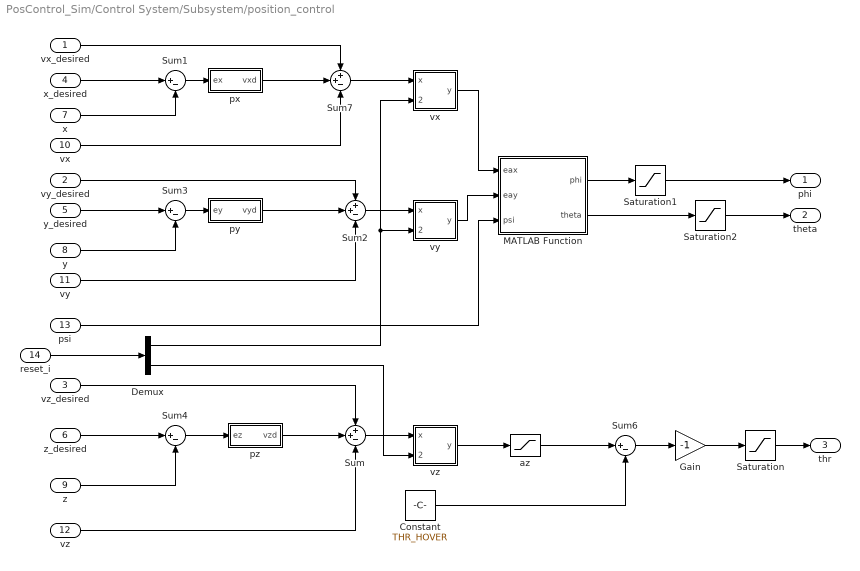
== system PosControl_Sim/Control System/Subsystem/position_control ==
  vx_desired : Inport
  vy_desired : Inport  Port=2
  vz_desired : Inport  Port=3
  x_desired : Inport  Port=4
  y_desired : Inport  Port=5
  z_desired : Inport  Port=6
  x : Inport  Port=7
  y : Inport  Port=8
  z : Inport  Port=9
  vx : Inport  Port=10
  vy : Inport  Port=11
  vz : Inport  Port=12
  psi : Inport  Port=13
  reset_i : Inport  Port=14
  Constant : Constant  Value=THR_HOVER
  Demux : Demux  Outputs=2
  Gain : Gain  Gain=-1
  MATLAB Function : MATLAB Function  TreatAsAtomicUnit=on
  Saturation : Saturate  UpperLimit=0.9  LowerLimit=0
  Saturation1 : Saturate  UpperLimit=MAX_CONTROL_ANGLE_ROLL*DEG2RAD  LowerLimit=-MAX_CONTROL_ANGLE_ROLL*DEG2RAD
  Saturation2 : Saturate  UpperLimit=MAX_CONTROL_ANGLE_PITCH*DEG2RAD/2  LowerLimit=-MAX_CONTROL_ANGLE_PITCH*DEG2RAD/2
  Sum : Sum  Inputs=++-
  Sum{1,3..4,6} (4 alike) : Sum  Inputs=|+-
  Sum2 : Sum  Inputs=++-
  Sum7 : Sum  Inputs=++-
  az : Saturate  UpperLimit=0.4  LowerLimit=-0.4
  px : Subsystem
  py : Subsystem
  pz : Subsystem
  "vx " : Subsystem
  "vy " : Subsystem
  "vz " : Subsystem
  phi : Outport
  theta : Outport  Port=2
  thr : Outport  Port=3
  wires:
  Saturation/1 -> thr/1
  Gain/1 -> Saturation/1
  Sum6/1 -> Gain/1
  "vz "/1(y) -> az/1
  Sum4/1 -> pz/1(ez)
  z/1 -> Sum4/2
  Constant/1 -> Sum6/2
  Sum/1 -> "vz "/1(x)
  vz/1 -> Sum/3
  vx/1 -> Sum7/3
  x/1 -> Sum1/2
  y/1 -> Sum3/2
  Sum3/1 -> py/1(ey)
  y_desired/1 -> Sum3/1
  vy/1 -> Sum2/3
  Sum2/1 -> "vy "/1(x)
  Sum7/1 -> "vx "/1(x)
  Sum1/1 -> px/1(ex)
  vy_desired/1 -> Sum2/1
  py/1(vyd) -> Sum2/2
  pz/1(vzd) -> Sum/2
  z_desired/1 -> Sum4/1
  vz_desired/1 -> Sum/1
  "vx "/1(y) -> MATLAB Function/1(eax)
  px/1(vxd) -> Sum7/2
  Saturation1/1 -> phi/1
  Saturation2/1 -> theta/1
  x_desired/1 -> Sum1/1
  vx_desired/1 -> Sum7/1
  "vy "/1(y) -> MATLAB Function/2(eay)
  psi/1 -> MATLAB Function/3(psi)
  MATLAB Function/1(phi) -> Saturation1/1
  MATLAB Function/2(theta) -> Saturation2/1
  reset_i/1 -> Demux/1
  Demux/1 -> "vy "/2(reset_i), "vx "/2(reset_i)
  Demux/2 -> "vz "/2(reset_i)
  az/1 -> Sum6/1

== system PosControl_Sim/Quadcopter Dynamics/Propulsor Model/Throttle To rads Gain _1 ==
  In5 : Inport
  Constant : Constant  Value=ModelParam_motorWb
  Gain : Gain  Gain=ModelParam_motorCr
  Sum1 : Sum  Inputs=++|
  Out5 : Outport
  wires:
  Constant/1 -> Sum1/1
  Gain/1 -> Sum1/2
  In5/1 -> Gain/1
  Sum1/1 -> Out5/1

== system PosControl_Sim/Quadcopter Dynamics/Propulsor Model/Throttle To rads Gain _2 ==
  In5 : Inport
  Constant : Constant  Value=ModelParam_motorWb
  Gain : Gain  Gain=ModelParam_motorCr
  Sum1 : Sum  Inputs=++|
  Out5 : Outport
  wires:
  Sum1/1 -> Out5/1
  In5/1 -> Gain/1
  Gain/1 -> Sum1/2
  Constant/1 -> Sum1/1

== system PosControl_Sim/Quadcopter Dynamics/Propulsor Model/Throttle To rads Gain _3 ==
  In5 : Inport
  Constant : Constant  Value=ModelParam_motorWb
  Gain : Gain  Gain=ModelParam_motorCr
  Sum1 : Sum  Inputs=++|
  Out5 : Outport
  wires:
  Constant/1 -> Sum1/1
  Gain/1 -> Sum1/2
  In5/1 -> Gain/1
  Sum1/1 -> Out5/1

== system PosControl_Sim/Quadcopter Dynamics/Propulsor Model/Throttle To rads Gain _4 ==
  In5 : Inport
  Constant : Constant  Value=ModelParam_motorWb
  Gain : Gain  Gain=ModelParam_motorCr
  Sum1 : Sum  Inputs=++|
  Out5 : Outport
  wires:
  Sum1/1 -> Out5/1
  In5/1 -> Gain/1
  Gain/1 -> Sum1/2
  Constant/1 -> Sum1/1

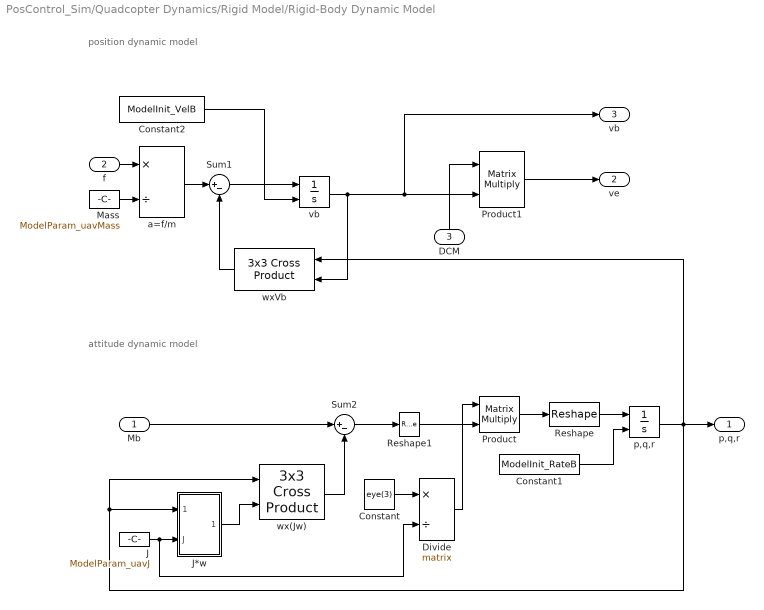
== system PosControl_Sim/Quadcopter Dynamics/Rigid Model/Rigid-Body Dynamic Model ==
  note: attitude dynamic model
  note: position dynamic model
  Mb : Inport
  f : Inport  Port=2
  DCM : Inport  Port=3
  " Mass " : Constant  Value=ModelParam_uavMass
  Constant : Constant  Value=eye(3)
  Constant1 : Constant  Value=ModelInit_RateB
  Constant2 : Constant  Value=ModelInit_VelB
  Divide : Product  Inputs=*/  Multiplication=Matrix(*)
  "J " : Constant  Value=ModelParam_uavJ
  J*w : Subsystem
  Product : Product  Multiplication=Matrix(*)
  Product1 : Product  Multiplication=Matrix(*)
  Reshape : Reshape  OutputDimensionality=Customize  OutputDimensions=[3,1]
  Reshape1 : Reshape  OutputDimensionality=Column vector (2-D)
  Sum1 : Sum  Inputs=|+-
  Sum2 : Sum  Inputs=|+-
  a=f/m : Product  Inputs=*/
  p,q,r : Integrator  InitialConditionSource=external
  vb : Integrator  InitialConditionSource=external
  wx(Jw) : sharedutil/3x3 Cross Product
      settings: SourceProductBaseCode=AE
  wxVb : sharedutil/3x3 Cross Product
      settings: SourceProductBaseCode=AE
  "p,q,r " : Outport
  ve : Outport  Port=2
  "vb " : Outport  Port=3
  wires:
  Product/1 -> Reshape/1
  Reshape1/1 -> Product/2
  Constant/1 -> Divide/1
  Divide/1 -> Product/1
  Sum2/1 -> Reshape1/1
  "J "/1 -> Divide/2, J*w/2(J)
  p,q,r/1 -> "p,q,r "/1, J*w/1(p q r), wx(Jw)/1, wxVb/1
  J*w/1("J*w ") -> wx(Jw)/2
  Mb/1 -> Sum2/1
  wx(Jw)/1 -> Sum2/2
  Constant2/1 -> vb/2
  f/1 -> a=f/m/1
  Product1/1 -> ve/1
  wxVb/1 -> Sum1/2
  a=f/m/1 -> Sum1/1
  Sum1/1 -> vb/1
  vb/1 -> Product1/2, "vb "/1, wxVb/2
  " Mass "/1 -> a=f/m/2
  DCM/1 -> Product1/1
  Reshape/1 -> p,q,r/1
  Constant1/1 -> p,q,r/2

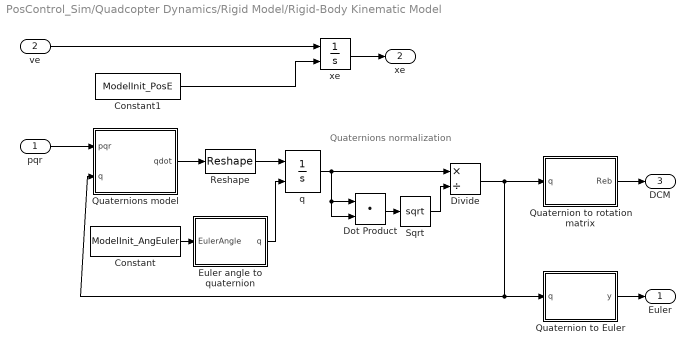
== system PosControl_Sim/Quadcopter Dynamics/Rigid Model/Rigid-Body Kinematic Model  ==
  note: Quaternions
      | normalization
  pqr : Inport
  ve : Inport  Port=2
  Constant : Constant  Value=ModelInit_AngEuler
  Constant1 : Constant  Value=ModelInit_PosE
  Divide : Product  Inputs=*/
  Dot Product : DotProduct  InputSameDT=on  OutDataTypeStr=Inherit: Inherit via internal rule
  Euler angle to quaternion : MATLAB Function
  Quaternion to Euler : MATLAB Function
  Quaternion to rotation matrix : MATLAB Function
  Quaternions model : MATLAB Function  TreatAsAtomicUnit=on
  Reshape : Reshape  OutputDimensionality=Customize  OutputDimensions=[4,1]
  Sqrt : Sqrt  SaturateOnIntegerOverflow=on
  q : Integrator  InitialConditionSource=external
  xe : Integrator  InitialConditionSource=external
  Euler : Outport
  "xe " : Outport  Port=2
  DCM : Outport  Port=3
  wires:
  Divide/1 -> Quaternion to rotation matrix/1(q), Quaternions model/2(q), Quaternion to Euler/1(q)
  Dot Product/1 -> Sqrt/1
  pqr/1 -> Quaternions model/1(pqr)
  q/1 -> Divide/1, Dot Product/1, Dot Product/2
  Quaternions model/1(qdot) -> Reshape/1
  Quaternion to rotation matrix/1(Reb) -> DCM/1
  Quaternion to Euler/1(y) -> Euler/1
  Constant/1 -> Euler angle to quaternion/1(EulerAngle)
  Euler angle to quaternion/1(q) -> q/2
  Reshape/1 -> q/1
  ve/1 -> xe/1
  xe/1 -> "xe "/1
  Constant1/1 -> xe/2
  Sqrt/1 -> Divide/2

== system PosControl_Sim/Control System/Subsystem/AttitudeControl/pitch_angle  ==
  x : Inport
  Gain : Gain  Gain=Kp_PITCH_ANGLE
  y : Outport  InitialOutput=0
  wires:
  x/1 -> Gain/1
  Gain/1 -> y/1

== system PosControl_Sim/Control System/Subsystem/AttitudeControl/pitch_rate ==
  x : Inport
  reset_i : Inport  Port=2
  Derivative Gain : Gain  DisableCoverage=on  Gain=Kd_PITCH_AngleRate  ParamMin=-100  ParamMax=100  OutMin=-100  OutMax=100
  Discrete Derivative : simulink/Discrete/Discrete Derivative  gainval=1.0  ICPrevScaledInput=0.0  OutMin=[]  OutMax=[]  OutDataType=fixdt(1, 16)  OutScaling=2^-10  DoSatur=off
  Discrete-Time Integrator : DiscreteIntegrator  ExternalReset=level  InitialConditionSetting=State (most efficient)  SampleTime=-1  LimitOutput=on  UpperSaturationLimit=Saturation_I_RP_Max  LowerSaturationLimit=Saturation_I_RP_Min  ICPrevOutput=DiscIntNeverNeededParam  ICPrevScaledInput=DiscIntNeverNeededParam
  Gain : Gain  Gain=Kp_PITCH_AngleRate
  Integral Gain : Gain  DisableCoverage=on  Gain=Ki_PITCH_AngleRate
  Sum : Sum  Inputs=+++
  y : Outport  InitialOutput=0
  wires:
  Discrete-Time Integrator/1 -> Sum/2
  Discrete Derivative/1 -> Sum/3
  Sum/1 -> y/1
  Gain/1 -> Sum/1
  Derivative Gain/1 -> Discrete Derivative/1
  Integral Gain/1 -> Discrete-Time Integrator/1
  x/1 -> Derivative Gain/1, Integral Gain/1, Gain/1
  reset_i/1 -> Discrete-Time Integrator/2

== system PosControl_Sim/Control System/Subsystem/AttitudeControl/roll_angle  ==
  x : Inport
  Gain : Gain  Gain=Kp_ROLL_ANGLE
  y : Outport  InitialOutput=0
  wires:
  Gain/1 -> y/1
  x/1 -> Gain/1

== system PosControl_Sim/Control System/Subsystem/AttitudeControl/roll_rate ==
  x : Inport
  reset_i : Inport  Port=2
  Derivative Gain : Gain  DisableCoverage=on  Gain=Kd_ROLL_AngleRate  ParamMin=-100  ParamMax=100  OutMin=-100  OutMax=100
  Discrete Derivative : simulink/Discrete/Discrete Derivative  gainval=1.0  ICPrevScaledInput=0.0  OutMin=[]  OutMax=[]  OutDataType=fixdt(1, 16)  OutScaling=2^-10  DoSatur=off
  Discrete-Time Integrator : DiscreteIntegrator  ExternalReset=level  InitialConditionSetting=State (most efficient)  SampleTime=-1  LimitOutput=on  UpperSaturationLimit=Saturation_I_RP_Max  LowerSaturationLimit=Saturation_I_RP_Min  ICPrevOutput=DiscIntNeverNeededParam  ICPrevScaledInput=DiscIntNeverNeededParam
  Gain : Gain  Gain=Kp_ROLL_AngleRate
  Integral Gain : Gain  DisableCoverage=on  Gain=Ki_ROLL_AngleRate
  Sum : Sum  Inputs=+++
  y : Outport  InitialOutput=0
  wires:
  x/1 -> Gain/1, Integral Gain/1, Derivative Gain/1
  Integral Gain/1 -> Discrete-Time Integrator/1
  Derivative Gain/1 -> Discrete Derivative/1
  Gain/1 -> Sum/1
  Sum/1 -> y/1
  Discrete Derivative/1 -> Sum/3
  Discrete-Time Integrator/1 -> Sum/2
  reset_i/1 -> Discrete-Time Integrator/2

== system PosControl_Sim/Control System/Subsystem/AttitudeControl/yaw_rate ==
  x : Inport
  reset_i : Inport  Port=2
  Derivative Gain : Gain  DisableCoverage=on  Gain=Kd_YAW_AngleRate  ParamMin=-100  ParamMax=100  OutMin=-100  OutMax=100
  Discrete Derivative : simulink/Discrete/Discrete Derivative  gainval=1.0  ICPrevScaledInput=0.0  OutMin=[]  OutMax=[]  OutDataType=fixdt(1, 16)  OutScaling=2^-10  DoSatur=off
  Discrete-Time Integrator : DiscreteIntegrator  ExternalReset=level  InitialConditionSetting=State (most efficient)  SampleTime=-1  LimitOutput=on  UpperSaturationLimit=Saturation_I_Y_Max  LowerSaturationLimit=Saturation_I_Y_Min  ICPrevOutput=DiscIntNeverNeededParam  ICPrevScaledInput=DiscIntNeverNeededParam
  Gain : Gain  Gain=Kp_YAW_AngleRate
  Integral Gain : Gain  DisableCoverage=on  Gain=Ki_YAW_AngleRate
  Sum : Sum  Inputs=+++
  y : Outport  InitialOutput=0
  wires:
  x/1 -> Gain/1, Integral Gain/1, Derivative Gain/1
  Integral Gain/1 -> Discrete-Time Integrator/1
  Derivative Gain/1 -> Discrete Derivative/1
  Gain/1 -> Sum/1
  Sum/1 -> y/1
  Discrete Derivative/1 -> Sum/3
  Discrete-Time Integrator/1 -> Sum/2
  reset_i/1 -> Discrete-Time Integrator/2

== system PosControl_Sim/Control System/Subsystem/position_control/px ==
  ex : Inport
  Gain1 : Gain  Gain=Kpxp
  Saturation3 : Saturate  UpperLimit=MAX_CONTROL_VELOCITY_XY  LowerLimit=-MAX_CONTROL_VELOCITY_XY
  vxd : Outport
  wires:
  ex/1 -> Gain1/1
  Saturation3/1 -> vxd/1
  Gain1/1 -> Saturation3/1

== system PosControl_Sim/Control System/Subsystem/position_control/py ==
  ey : Inport
  Gain1 : Gain  Gain=Kpyp
  Saturation3 : Saturate  UpperLimit=MAX_CONTROL_VELOCITY_XY  LowerLimit=-MAX_CONTROL_VELOCITY_XY
  vyd : Outport
  wires:
  Gain1/1 -> Saturation3/1
  Saturation3/1 -> vyd/1
  ey/1 -> Gain1/1

== system PosControl_Sim/Control System/Subsystem/position_control/pz ==
  ez : Inport
  Gain1 : Gain  Gain=Kpzp
  Saturation3 : Saturate  UpperLimit=MAX_CONTROL_VELOCITY_Z  LowerLimit=-MAX_CONTROL_VELOCITY_Z
  vzd : Outport
  wires:
  ez/1 -> Gain1/1
  Saturation3/1 -> vzd/1
  Gain1/1 -> Saturation3/1

== system PosControl_Sim/Control System/Subsystem/position_control/vx  ==
  x : Inport
  reset_i : Inport  Port=2
  Derivative Gain : Gain  DisableCoverage=on  Gain=Kvxd
  Discrete Derivative : simulink/Discrete/Discrete Derivative  gainval=1.0  ICPrevScaledInput=0.0  OutMin=[]  OutMax=[]  OutDataType=fixdt(1, 16)  OutScaling=2^-10  DoSatur=off
  Discrete-Time Integrator : DiscreteIntegrator  ExternalReset=level  InitialConditionSetting=State (most efficient)  SampleTime=-1  LimitOutput=on  UpperSaturationLimit=Saturation_I_ah  LowerSaturationLimit=-Saturation_I_ah  ICPrevOutput=DiscIntNeverNeededParam  ICPrevScaledInput=DiscIntNeverNeededParam
  Gain : Gain  Gain=Kvxp
  Integral Gain : Gain  DisableCoverage=on  Gain=Kvxi
  Sum : Sum  Inputs=+++
  y : Outport  InitialOutput=0
  wires:
  x/1 -> Gain/1, Integral Gain/1, Derivative Gain/1
  Integral Gain/1 -> Discrete-Time Integrator/1
  Derivative Gain/1 -> Discrete Derivative/1
  Gain/1 -> Sum/1
  Sum/1 -> y/1
  Discrete Derivative/1 -> Sum/3
  Discrete-Time Integrator/1 -> Sum/2
  reset_i/1 -> Discrete-Time Integrator/2

== system PosControl_Sim/Control System/Subsystem/position_control/vy  ==
  x : Inport
  reset_i : Inport  Port=2
  Derivative Gain : Gain  DisableCoverage=on  Gain=Kvyd
  Discrete Derivative : simulink/Discrete/Discrete Derivative  gainval=1.0  ICPrevScaledInput=0.0  OutMin=[]  OutMax=[]  OutDataType=fixdt(1, 16)  OutScaling=2^-10  DoSatur=off
  Discrete-Time Integrator : DiscreteIntegrator  ExternalReset=level  InitialConditionSetting=State (most efficient)  SampleTime=-1  LimitOutput=on  UpperSaturationLimit=Saturation_I_ah  LowerSaturationLimit=-Saturation_I_ah  ICPrevOutput=DiscIntNeverNeededParam  ICPrevScaledInput=DiscIntNeverNeededParam
  Gain : Gain  Gain=Kvyp
  Integral Gain : Gain  DisableCoverage=on  Gain=Kvyi
  Sum : Sum  Inputs=+++
  y : Outport  InitialOutput=0
  wires:
  x/1 -> Gain/1, Integral Gain/1, Derivative Gain/1
  Integral Gain/1 -> Discrete-Time Integrator/1
  Derivative Gain/1 -> Discrete Derivative/1
  Gain/1 -> Sum/1
  Sum/1 -> y/1
  Discrete Derivative/1 -> Sum/3
  Discrete-Time Integrator/1 -> Sum/2
  reset_i/1 -> Discrete-Time Integrator/2

== system PosControl_Sim/Control System/Subsystem/position_control/vz  ==
  x : Inport
  reset_i : Inport  Port=2
  Derivative Gain : Gain  DisableCoverage=on  Gain=Kvzd
  Discrete Derivative : simulink/Discrete/Discrete Derivative  gainval=1.0  ICPrevScaledInput=0.0  OutMin=[]  OutMax=[]  OutDataType=fixdt(1, 16)  OutScaling=2^-10  DoSatur=off
  Discrete-Time Integrator : DiscreteIntegrator  ExternalReset=level  InitialConditionSetting=State (most efficient)  SampleTime=-1  LimitOutput=on  UpperSaturationLimit=Saturation_I_az  LowerSaturationLimit=-Saturation_I_az  ICPrevOutput=DiscIntNeverNeededParam  ICPrevScaledInput=DiscIntNeverNeededParam
  Gain : Gain  Gain=Kvzp
  Integral Gain : Gain  DisableCoverage=on  Gain=Kvzi
  Sum : Sum  Inputs=+++
  y : Outport  InitialOutput=0
  wires:
  Discrete-Time Integrator/1 -> Sum/2
  Discrete Derivative/1 -> Sum/3
  Sum/1 -> y/1
  Gain/1 -> Sum/1
  Derivative Gain/1 -> Discrete Derivative/1
  Integral Gain/1 -> Discrete-Time Integrator/1
  x/1 -> Derivative Gain/1, Integral Gain/1, Gain/1
  reset_i/1 -> Discrete-Time Integrator/2

== system PosControl_Sim/Quadcopter Dynamics/Rigid Model/Rigid-Body Dynamic Model/J*w ==
  p q r : Inport
  J : Inport  Port=2
  J*w : Product  Multiplication=Matrix(*)
  "J*w " : Outport
  wires:
  J*w/1 -> "J*w "/1
  J/1 -> J*w/1
  p q r/1 -> J*w/2

== matlab function PosControl_Sim/Control System/MATLAB Function1 ==
  data: reset_i output; ch3 input
function reset_i= fcn(ch3)
%Function description:
%  Reset Integral when throttle < 1250
if ch3<1250
    reset_i=[1 1 1 1];
else
    reset_i=[0 0 0 0];
end

== matlab function PosControl_Sim/Control System/InputConditioning/deadzone2 ==
  data: u input; y output
function y = fcn(u)
%Function description:
%  Control the range of the remote control input from RCMin to RCMax, and
%  set a dead zone with a dead zone size of ±deadZone. The output y is
%  normalized to 0~1.You can get the RC calibration parameters in QGC.
RCMin = 1100;
RCMax = 1900;
RCMid = (RCMin + RCMax)/2;
deadZoneRate = 0.05;
deadZone = deadZoneRate*(RCMax - RCMin);
k = 1/(RCMax - RCMid - deadZone);
% saturation
if(u < RCMin)
    u = RCMin;
elseif(u > RCMax)
    u = RCMax;
end
% dead zone and normalize
 if(u > RCMid + deadZone)
    y = (u-RCMid - deadZone)*k;
 elseif(u < RCMid - deadZone)
     y = (u - RCMid + deadZone)*k;
 else
     y = 0;
 end

 end

== matlab function PosControl_Sim/Control System/InputConditioning/deadzone1 ==
  data: u input; y output
function y = fcn(u)
%Function description:
%  Control the range of the remote control input from RCMin to RCMax, and
%  set a dead zone with a dead zone size of ±deadZone. The output y is
%  normalized to 0~1.You can get the RC calibration parameters in QGC.
RCMin = 1100;
RCMax = 1900;
RCMid = (RCMin + RCMax)/2;
deadZoneRate = 0.05;
deadZone = deadZoneRate*(RCMax - RCMin);
k = 1/(RCMax - RCMid - deadZone);
% saturation
if(u < RCMin)
    u = RCMin;
elseif(u > RCMax)
    u = RCMax;
end
% dead zone and normalize
 if(u > RCMid + deadZone)
    y = (u-RCMid - deadZone)*k;
 elseif(u < RCMid - deadZone)
     y = (u - RCMid + deadZone)*k;
 else
     y = 0;
 end

 end

== matlab function PosControl_Sim/Control System/InputConditioning1/deadzone1 ==
  data: u input; y output
function y = fcn(u)
%Function description:
%  Control the range of the remote control input from RCMin to RCMax, and
%  set a dead zone with a dead zone size of ±deadZone. The output y is
%  normalized to 0~1.You can get the RC calibration parameters in QGC.
RCMin = 1100;
RCMax = 1900;
RCMid = (RCMin + RCMax)/2;
deadZoneRate = 0.05;
deadZone = deadZoneRate*(RCMax - RCMin);
k = 1/(RCMax - RCMid - deadZone);
% saturation
if(u < RCMin)
    u = RCMin;
elseif(u > RCMax)
    u = RCMax;
end
% dead zone and normalize
 if(u > RCMid + deadZone)
    y = (u-RCMid - deadZone)*k;
 elseif(u < RCMid - deadZone)
     y = (u - RCMid + deadZone)*k;
 else
     y = 0;
 end

 end

== matlab function PosControl_Sim/Control System/InputConditioning1/deadzone2 ==
  data: u input; y output
function y = fcn(u)
%Function description:
%  Control the range of the remote control input from RCMin to RCMax, and
%  set a dead zone with a dead zone size of ±deadZone. The output y is
%  normalized to 0~1.You can get the RC calibration parameters in QGC.
RCMin = 1100;
RCMax = 1900;
RCMid = (RCMin + RCMax)/2;
deadZoneRate = 0.05;
deadZone = deadZoneRate*(RCMax - RCMin);
k = 1/(RCMax - RCMid - deadZone);
% saturation
if(u < RCMin)
    u = RCMin;
elseif(u > RCMax)
    u = RCMax;
end
% dead zone and normalize
 if(u > RCMid + deadZone)
    y = (u-RCMid - deadZone)*k;
 elseif(u < RCMid - deadZone)
     y = (u - RCMid + deadZone)*k;
 else
     y = 0;
 end

 end

== matlab function PosControl_Sim/Control System/InputConditioning1/deadzone3 ==
  data: u input; y output
function y = fcn(u)
%Function description:
%  Control the range of the remote control input from RCMin to RCMax, and
%  set a dead zone with a dead zone size of ±deadZone. The output y is
%  normalized to 0~1.You can get the RC calibration parameters in QGC.
RCMin = 1100;
RCMax = 1900;
RCMid = (RCMin + RCMax)/2;
deadZoneRate = 0.05;
deadZone = deadZoneRate*(RCMax - RCMin);
k = 1/(RCMax - RCMid - deadZone);
% saturation
if(u < RCMin)
    u = RCMin;
elseif(u > RCMax)
    u = RCMax;
end
% dead zone and normalize
 if(u > RCMid + deadZone)
    y = (u-RCMid - deadZone)*k;
 elseif(u < RCMid - deadZone)
     y = (u - RCMid + deadZone)*k;
 else
     y = 0;
 end

 end

== matlab function PosControl_Sim/Control System/InputConditioning/deadzone3 ==
  data: u input; y output
function y = fcn(u)
%Function description:
%  Control the range of the remote control input from RCMin to RCMax, and
%  set a dead zone with a dead zone size of ±deadZone. The output y is
%  normalized to 0~1.You can get the RC calibration parameters in QGC.
RCMin = 1100;
RCMax = 1900;
RCMid = (RCMin + RCMax)/2;
deadZoneRate = 0.05;
deadZone = deadZoneRate*(RCMax - RCMin);
k = 1/(RCMax - RCMid - deadZone);
% saturation
if(u < RCMin)
    u = RCMin;
elseif(u > RCMax)
    u = RCMax;
end
% dead zone and normalize
 if(u > RCMid + deadZone)
    y = (u-RCMid - deadZone)*k;
 elseif(u < RCMid - deadZone)
     y = (u - RCMid + deadZone)*k;
 else
     y = 0;
 end

 end

== matlab function PosControl_Sim/Control System/MATLAB Function2 ==
  settings: updateMethod=DISCRETE
  data: vxd input; vyd input; vx_d output; vy_d output; vz_d output; vzd input; x input; y input; z input; vx input; vy input; vz input; x_d output; y_d output; z_d output
function [vx_d, vy_d, vz_d, x_d, y_d, z_d]  = fcn(vxd, vyd, vzd, x, y, z, vx, vy, vz)
%Function description:
%  position control implementation. When the desired velocity (specified by the remote controller) is < 0.001, 
%  and the current velocity is <6 m/s, the position hold is activated, and the desired position is the position at which 
%  the above condition is satisfied, the position loop and the velocity loop act simultaneously; when the condition 
%  is not satisfied, Only the velocity loop works.
%Input:
%  vxd, vyd, vzd: The desired velocity specified by the remote control
%  x, y, z: current position
%  vx, vy,vz: current velocity
%Output:
%  vx_d, vy_d, vz_d, x_d, y_d, z_d: desired velocity and position
persistent x1;
if isempty(x1)
    x1 = 0;
end
persistent y1;
if isempty(y1)
    y1 = 0;
end
persistent z1;
if isempty(z1)
    z1 = z;
end
persistent hold_x_flag;
if isempty(hold_x_flag)
    hold_x_flag = 0;
end
persistent hold_y_flag;
if isempty(hold_y_flag)
    hold_y_flag = 0;
end
persistent hold_z_flag;
if isempty(hold_z_flag)
    hold_z_flag = 0;
end

if abs(vxd) < 0.001 && abs(vx) < 8
    hold_x = 1;
else
    hold_x = 0;
    hold_x_flag = 0;
end
if abs(vyd) < 0.001 && abs(vy) < 8
    hold_y = 1;
else
    hold_y = 0;
    hold_y_flag = 0;
end
if abs(vzd) < 0.001 && abs(vz) < 6
    hold_z = 1;
else
    hold_z = 0;
    hold_z_flag = 0;
end

if (hold_x > 0.5) && (hold_x_flag < 0.5)
    x1 = x;
    hold_x_flag = 1;
end
if (hold_y > 0.5) && (hold_y_flag < 0.5)
    y1 = y;
    hold_y_flag = 1;
end

% throttle in the middle position, hold the height
if (hold_z > 0.5) && (hold_z_flag < 0.5)
    z1 = z;
    hold_z_flag = 1;
end
%When the RC sticks(CH1, CH2, CH3, CH4) deviate from the middle dead zone range, the position is the current position. 
%The position controller only works with the velocity loop
if hold_x < 0.5
    x1 = x;
    hold_x_flag = 0;
end
if hold_y < 0.5
    y1 = y;
    hold_y_flag = 0;
end
if hold_z < 0.5
    z1 = z;
    hold_z_flag = 0;
end
vx_d = vxd; vy_d = vyd; vz_d = vzd;

x_d = x1;
y_d = y1;
z_d = z1;

== matlab function PosControl_Sim/Control System/Subsystem/position_control/MATLAB Function ==
  data: eax input; eay input; psi input; phi output; theta output
function [phi, theta] = fcn(eax, eay, psi)
%Function description:
%  Convert the desired horizontal acceleration to the desired attitude angle
%Input:
%  eax, eaxy: desired horizontal acceleration
%  psi: yaw
%Output:
%  phi, theta: desired roll angle and desired pitch angle
g = 9.8;
phi = (-sin(psi)*eax + cos(psi)*eay)/g;
theta = (-cos(psi)*eax - sin(psi)*eay)/g;
